simulink model "Deskrealtime"  (R2019b)
settings: Solver=FixedStepDiscrete  StartTime=0.0  StopTime=200  FixedStep=0.1  RelTol=1e-3  AbsTol=1e-6
model workspace (MATLAB code in the model file + MAT data in the model file):
  | Ts=0.1;
undefined symbols (not defined in the file or in its folder): National_Instruments, PCIe, sldrtexcb_modeswitch
libraries: xpcseriallib x60, sldrtlib x6, xpcrtudplib x2
Description:
  | Frequency Measurement
  | 
  | The example model "sldrtex_counter" shows how to measure input signal frequency using
  | Simulink Desktop Real-Time(TM). The measured signal is connected to the counter
  | input of your data acquisition board. Counter Input block is configured
  | to reset counter each sample-hit after counter read. Dividing counter
  | value by sample time gives input signal frequency.
  | 
  | How to run this model in Normal Mode:
  | 
  | 1) Open the Counter Input block and select your data acquisition board.
  |    If there's no board installed, install it using the Install new board button.
  | 2) Double-click the orange button to switch to Normal Mode if needed.
  | 3) Start the real-time execution using Simulation->Run.
  | 
  | How to run this model in External Mode:
  | 
  | 1) Open the Counter Input block and select your data acquisition board.
  |    If there's no board installed, install it using the Install new board button.
  | 2) Double-click the orange button to switch to External Mode if needed.
  | 3) Start the real-time execution using Simulation->Run. The model will automatically
  |    build, connect to Simulink in External Mode and start.
  | 
  | Note: To run this model, you must have a data acquisition board with counter input
  |    connected to your computer.
settings Model: xpc_rtwmakecfg_data=_xpcnblib__xpcetherlib__xpcether8255xlib__xpcetherGbElib__xpciplib_  PacingRate=0.400000  Creator=The MathWorks, Inc.  LastModifiedBy=qzlab
settings SolverCC: AutoScaleAbsTol=off
settings DataIOCC: ExternalInput=[]  InitialState=[]  MaxDataPoints=5000  SaveFormat=Array  SaveOutput=off  SaveTime=off  ReturnWorkspaceOutputs=off  SignalLoggingName=sigsOut
settings OptimizationCC: BlockReduction=off  BooleanDataType=off  ExpressionDepthLimit=2147483647  InitFltsAndDblsToZero=on  EfficientMapNaN2IntZero=off  LifeSpan=inf
settings DebuggingCC: UnderspecifiedInitializationDetection=Classic  MergeDetectMultiDrivingBlocksExec=none  SignalResolutionControl=TryResolveAllWithWarning  MultiTaskDSMMsg=warning  MultiTaskCondExecSysMsg=none  IntegerOverflowMsg=none  FcnCallInpInsideContextMsg=warning  AllowSymbolicDim=off  StateNameClashWarn=warning  SymbolicDimsDataTypeCodeGenerationDiagnostic=none  SFUnexpectedBacktrackingDiag=warning  SFNoUnconditionalDefaultTransitionDiag=warning  SFExecutionAtInitializationDiag=none  IntegerSaturationMsg=none  ArithmeticOperatorsInVariantConditions=warning
settings HardwareCC: TargetBitPerLong=64  TargetBitPerPointer=64  TargetBitPerSizeT=64  TargetBitPerPtrDiffT=64  TargetIntDivRoundTo=Zero  TargetEndianess=LittleEndian  TargetWordSize=64  TargetHWDeviceType=Intel->x86-64
settings ModelReferenceCC: PropagateSignalLabelsOutOfModel=off
settings SFSimCC: SimUseLocalCustomCode=off
settings RTWCC: Description=Simulink Desktop Real-Time  SystemTargetFile=sldrt.tlc  TemplateMakefile=sldrt.tmf  RTWUseLocalCustomCode=off  RTWCompilerOptimization=on
settings CodeAppCC: MaxIdLength=95  StateflowObjectComments=on
settings SimulinkDesktopRealTimeCC: TargetPreCompLibLocation=C:\Matalb2019B\toolbox\sldrt\lib\win64  TargetLangStandard=C89/C90 (ANSI)  GeneratePreprocessorConditionals=Disable all  SupportVariableSizeSignals=off  PreserveStateflowLocalDataDimensions=off
settings ConfigComp: CovMetricSettings=d  CovHtmlReporting=on  CovSaveCumulativeToWorkspaceVar=on  CovSaveSingleToWorkspaceVar=on  CovShowResultsExplorer=off  CovExternalEMLEnable=off  CovSFcnEnable=off

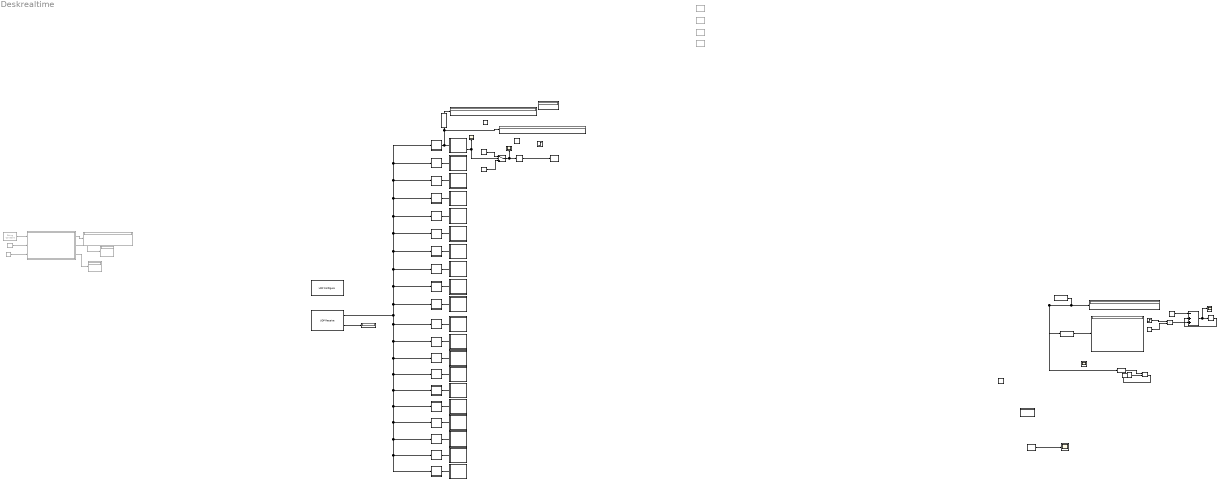
== system Deskrealtime ==
  note: Copyright 1994-2019 The MathWorks, Inc.
  note: To run the example in Normal mode, use the SIMULATION tab.
      | To run the example in External mode, use the DESKTOP REAL-TIME tab.
  1 : Subsystem
  10 : Subsystem
  11 : Subsystem
  12 : Subsystem
  13 : Subsystem
  14 : Subsystem
  15 : Subsystem
  16 : Subsystem
  17 : Subsystem
  18 : Subsystem
  19 : Subsystem
  2 : Subsystem
  2-1 : Subsystem
  2-10 : Subsystem
  2-11 : Subsystem
  2-12 : Subsystem
  2-13 : Subsystem
  2-14 : Subsystem
  2-15 : Subsystem
  2-16 : Subsystem
  2-17 : Subsystem
  2-18 : Subsystem
  2-19 : Subsystem
  2-2 : Subsystem
  2-20 : Subsystem
  2-3 : Subsystem
  2-4 : Subsystem
  2-5 : Subsystem
  2-6 : Subsystem
  2-7 : Subsystem
  2-8 : Subsystem
  2-9 : Subsystem
  20 : Subsystem
  3 : Subsystem
  4 : Subsystem
  5 : Subsystem
  6 : Subsystem
  7 : Subsystem
  8 : Subsystem
  9 : Subsystem
  ASCII to String : ASCIIToString
  ASCII to String1 : ASCIIToString
  Add : Sum  Inputs=-++
  Constant : Constant  Value=0
  Constant1 : Constant  Value=0
  Constant2 : Constant
  Constant3 : Constant
  Constant5 : Constant  Value=6  OutDataTypeStr=uint32
  Constant6 : Constant  Commented=on  Value=3  OutDataTypeStr=uint32
  Constant7 : Constant  Commented=on  OutDataTypeStr=uint32
  Constant8 : Constant
  Constant9 : Constant  Value=3
  Data Store Memory : DataStoreMemory  ReadBeforeWriteMsg=warning  WriteAfterWriteMsg=warning  WriteAfterReadMsg=warning  ShowAdditionalParam=off  OutDataTypeStr=uint32
  Data Store Write : DataStoreWrite
  Delay : Delay  DelayLength=1  InitialCondition=0
  Digital Output : sldrtlib/Digital Output  SampleTime=0.1  MaxMissedTicks=10  ShowMissedTicks=off  YieldWhenWaiting=off  DrvName=National_Instruments/PCIe-6259  DrvAddress=4294967295  DrvOptions=[0 2097151 65535 0 0]  Channels=[18:20]  BitMode=1  InitialValue=[]  FinalValue=[]
      settings: AttributesFormatString=National Instruments\nPCIe-6259 [auto]  SourceProductName=Simulink Desktop Real-Time  SourceProductBaseCode=WT
  Digital Output{1..4} (4 alike) : sldrtlib/Digital Output  Commented=on  SampleTime=0.1  MaxMissedTicks=10  ShowMissedTicks=off  YieldWhenWaiting=off  DrvName=National_Instruments/PCIe-6259  DrvAddress=4294967295  DrvOptions=[0 2097151 65535 0 0]  Channels=[19:20]  BitMode=1  InitialValue=[]  FinalValue=[]
      settings: AttributesFormatString=National Instruments\nPCIe-6259 [auto]  SourceProductName=Simulink Desktop Real-Time  SourceProductBaseCode=WT
  Display{1..3,6,8,10} (6 alike) : Display
  Display11 : Display  Commented=on
  Display12 : Display  Commented=on
  Display14 : Display  Commented=on
  Divide : Product  Inputs=*/  OutDataTypeStr=uint32
  Info : Subsystem  InitFcn=sldrtexcb_modeswitch('CheckKernel');  mask(Simulink Desktop Real-Time Example Info){}
      settings: OpenFcn=helpview([docroot '/sldrt/helptargets.map'], 'FrequencyMeasurementExample')
      mask Display: disp('Info')
  Missed Ticks : Scope
  Product : Product
  Real-Time Synchronization : sldrtlib/Real-Time Synchronization  SampleTime=0.1  MaxMissedTicks=Inf  ShowMissedTicks=on  YieldWhenWaiting=off
  Scope{,1..3} (4 alike) : Scope
  Step : Step  Time=0.01  Before=1  After=0
  Step1 : Step
  String Constant1 : StringConstant  Commented=on  String="\"123456789\""
  String Length1 : StringLength
  String to ASCII : StringToASCII
  Switch : Switch  Criteria=u2 > Threshold  Threshold=0.5
  Transport Delay : TransportDelay  DelayTime=10  InitialOutput=1
  UDP Configure : xpcrtudplib/UDP Configure  Priority=-1  IpAddress=127.0.0.1  SubnetMask=255.255.255.0  Gateway=0.0.0.0  PciBus=[2]  PciSlot=[0]  PciFunction=0  ID=1  tune=0  disable=off  enableMulticast=off  MulticastIpAddress={}  MulticastMask={}
      settings: SourceProductName=Simulink Real-Time  SourceProductBaseCode=XP
  UDP Receive2 : xpcrtudplib/UDP Receive  ipAddressVal=127.0.0.1  localPort=8001  rcvWidth=200  rcvFmAny=on  fmAddress=0.0.0.0  rcvMulticast=off  multicastAddress={}  maxUDPQueue=8  sampleTime=0.1
      settings: SourceProductName=Simulink Real-Time
  While Iterator Subsystem1 : Subsystem  Commented=on  TreatAsAtomicUnit=on
  wires:
  ASCII to String1/1 -> String to ASCII/1, String Length1/1, Display8/1
  String Length1/1 -> Divide/1
  Divide/1 -> Data Store Write/1
  Constant5/1 -> Divide/2
  String to ASCII/1 -> Display10/1
  String Constant1/1 -> While Iterator Subsystem1/1(In1)
  Constant6/1 -> While Iterator Subsystem1/2(In2)
  Constant7/1 -> While Iterator Subsystem1/3(In3)
  While Iterator Subsystem1/2(Out2) -> Display12/1
  While Iterator Subsystem1/1(Out1) -> Display11/1
  Product/1 -> Add/3
  Delay/1 -> Add/2
  Add/1 -> Scope2/1, Delay/1
  Constant8/1 -> Add/1
  Step/1 -> Product/1
  Constant9/1 -> Product/2
  While Iterator Subsystem1/3(Out3) -> Display14/1
  UDP Receive2/2 -> Display1/1
  Real-Time Synchronization/1 -> Missed Ticks/1
  UDP Receive2/1 -> 20/1(In1), 19/1(In1), 18/1(In1), 17/1(In1), 16/1(In1), 15/1(In1), 14/1(In1), 13/1(In1), 12/1(In1), 11/1(In1), 10/1(In1), 9/1(In1), 8/1(In1), 7/1(In1), 6/1(In1), 5/1(In1), 4/1(In1), 3/1(In1), 2/1(In1), 1/1(In1)
  3/1(Out1) -> 2-3/1(In1)
  2/1(Out1) -> 2-2/1(In1)
  4/1(Out1) -> 2-4/1(In1)
  5/1(Out1) -> 2-5/1(In1)
  6/1(Out1) -> 2-6/1(In1)
  7/1(Out1) -> 2-7/1(In1)
  8/1(Out1) -> 2-8/1(In1)
  9/1(Out1) -> 2-9/1(In1)
  10/1(Out1) -> 2-10/1(In1)
  11/1(Out1) -> 2-11/1(In1)
  12/1(Out1) -> 2-12/1(In1)
  13/1(Out1) -> 2-13/1(In1)
  14/1(Out1) -> 2-14/1(In1)
  15/1(Out1) -> 2-15/1(In1)
  16/1(Out1) -> 2-16/1(In1)
  17/1(Out1) -> 2-17/1(In1)
  18/1(Out1) -> 2-18/1(In1)
  19/1(Out1) -> 2-19/1(In1)
  20/1(Out1) -> 2-20/1(In1)
  2-1/3(Property) -> Scope3/1, Switch/2
  ASCII to String/1 -> Display2/1
  1/1(Out1) -> 2-1/1(In1), Display3/1, ASCII to String/1
  Constant1/1 -> Switch/1
  Switch/1 -> Transport Delay/1, Scope1/1
  Constant3/1 -> Switch/3
  Transport Delay/1 -> Digital Output/1

== system Deskrealtime/1 ==
  In1 : Inport
  ASCII to String : ASCIIToString  Commented=on
  Constant1 : Constant  Value=[1:9]
  Selector : Selector  InputPortWidth=200  IndexOptions=Index vector (port)  Indices=[1 3]  OutputSizes=1
  Out1 : Outport
  wires:
  Constant1/1 -> Selector/2
  In1/1 -> Selector/1
  Selector/1 -> Out1/1

== system Deskrealtime/10 ==
  In1 : Inport
  Constant1 : Constant  Value=[80:88]
  Selector : Selector  InputPortWidth=200  IndexOptions=Index vector (port)  Indices=[1 3]  OutputSizes=1
  Out1 : Outport
  wires:
  Constant1/1 -> Selector/2
  In1/1 -> Selector/1
  Selector/1 -> Out1/1

== system Deskrealtime/11 ==
  In1 : Inport
  Constant1 : Constant  Value=[89:89+8]
  Selector : Selector  InputPortWidth=200  IndexOptions=Index vector (port)  Indices=[1 3]  OutputSizes=1
  Out1 : Outport
  wires:
  Constant1/1 -> Selector/2
  In1/1 -> Selector/1
  Selector/1 -> Out1/1

== system Deskrealtime/12 ==
  In1 : Inport
  Constant1 : Constant  Value=[97:97+8]
  Selector : Selector  InputPortWidth=200  IndexOptions=Index vector (port)  Indices=[1 3]  OutputSizes=1
  Out1 : Outport
  wires:
  Constant1/1 -> Selector/2
  In1/1 -> Selector/1
  Selector/1 -> Out1/1

== system Deskrealtime/13 ==
  In1 : Inport
  Constant1 : Constant  Value=[105:105+8]
  Selector : Selector  InputPortWidth=200  IndexOptions=Index vector (port)  Indices=[1 3]  OutputSizes=1
  Out1 : Outport
  wires:
  Constant1/1 -> Selector/2
  In1/1 -> Selector/1
  Selector/1 -> Out1/1

== system Deskrealtime/14 ==
  In1 : Inport
  Constant1 : Constant  Value=[114:122]
  Selector : Selector  InputPortWidth=200  IndexOptions=Index vector (port)  Indices=[1 3]  OutputSizes=1
  Out1 : Outport
  wires:
  Constant1/1 -> Selector/2
  In1/1 -> Selector/1
  Selector/1 -> Out1/1

== system Deskrealtime/15 ==
  In1 : Inport
  Constant1 : Constant  Value=[123:123+8]
  Selector : Selector  InputPortWidth=200  IndexOptions=Index vector (port)  Indices=[1 3]  OutputSizes=1
  Out1 : Outport
  wires:
  Selector/1 -> Out1/1
  In1/1 -> Selector/1
  Constant1/1 -> Selector/2

== system Deskrealtime/16 ==
  In1 : Inport
  Constant1 : Constant  Value=[132:132+8]
  Selector : Selector  InputPortWidth=200  IndexOptions=Index vector (port)  Indices=[1 3]  OutputSizes=1
  Out1 : Outport
  wires:
  Selector/1 -> Out1/1
  In1/1 -> Selector/1
  Constant1/1 -> Selector/2

== system Deskrealtime/17 ==
  In1 : Inport
  Constant1 : Constant  Value=[141:141+8]
  Selector : Selector  InputPortWidth=200  IndexOptions=Index vector (port)  Indices=[1 3]  OutputSizes=1
  Out1 : Outport
  wires:
  Constant1/1 -> Selector/2
  In1/1 -> Selector/1
  Selector/1 -> Out1/1

== system Deskrealtime/18 ==
  In1 : Inport
  Constant1 : Constant  Value=[150:158]
  Selector : Selector  InputPortWidth=200  IndexOptions=Index vector (port)  Indices=[1 3]  OutputSizes=1
  Out1 : Outport
  wires:
  Selector/1 -> Out1/1
  In1/1 -> Selector/1
  Constant1/1 -> Selector/2

== system Deskrealtime/19 ==
  In1 : Inport
  Constant1 : Constant  Value=[159:159+8]
  Selector : Selector  InputPortWidth=200  IndexOptions=Index vector (port)  Indices=[1 3]  OutputSizes=1
  Out1 : Outport
  wires:
  Constant1/1 -> Selector/2
  In1/1 -> Selector/1
  Selector/1 -> Out1/1

== system Deskrealtime/2 ==
  In1 : Inport
  ASCII to String : ASCIIToString  Commented=on
  Constant1 : Constant  Value=[10:18]
  Selector : Selector  InputPortWidth=200  IndexOptions=Index vector (port)  Indices=[1 3]  OutputSizes=1
  Out1 : Outport
  wires:
  Constant1/1 -> Selector/2
  In1/1 -> Selector/1
  Selector/1 -> Out1/1

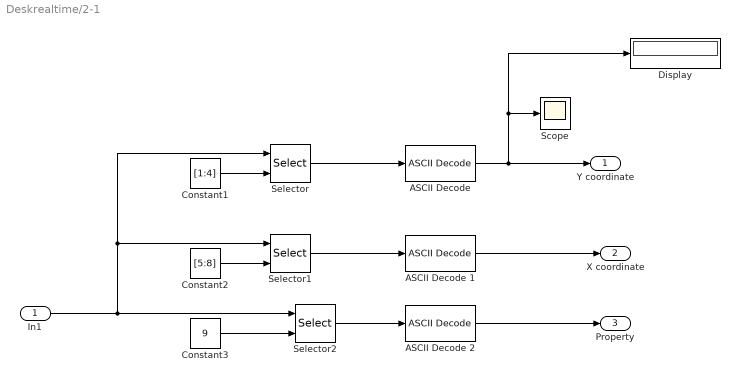
== system Deskrealtime/2-1 ==
  In1 : Inport
  "ASCII Decode " : xpcseriallib/ASCII Decode   format=%d\r  nvars=1  vartypes={ }
      settings: SourceProductName=Simulink Real-Time  SourceProductBaseCode=XP
  ASCII Decode 1 : xpcseriallib/ASCII Decode   format=%d\r  nvars=1  vartypes={ }
      settings: SourceProductName=Simulink Real-Time  SourceProductBaseCode=XP
  ASCII Decode 2 : xpcseriallib/ASCII Decode   format=%d\r  nvars=1  vartypes={ }
      settings: SourceProductName=Simulink Real-Time  SourceProductBaseCode=XP
  Constant1 : Constant  Value=[1:4]
  Constant2 : Constant  Value=[5:8]
  Constant3 : Constant  Value=9
  Display : Display
  Scope : Scope
  Selector : Selector  InputPortWidth=9  IndexOptions=Index vector (port)  Indices=[1 3]  OutputSizes=1
  Selector1 : Selector  InputPortWidth=9  IndexOptions=Index vector (port)  Indices=[1 3]  OutputSizes=1
  Selector2 : Selector  InputPortWidth=9  IndexOptions=Index vector (port)  Indices=[1 3]  OutputSizes=1
  Y coordinate : Outport
  X coordinate : Outport  Port=2
  Property : Outport  Port=3
  wires:
  Constant1/1 -> Selector/2
  In1/1 -> Selector2/1, Selector1/1, Selector/1
  Selector/1 -> "ASCII Decode "/1
  Constant2/1 -> Selector1/2
  Constant3/1 -> Selector2/2
  Selector1/1 -> ASCII Decode 1/1
  Selector2/1 -> ASCII Decode 2/1
  ASCII Decode 1/1 -> X coordinate/1
  ASCII Decode 2/1 -> Property/1
  "ASCII Decode "/1 -> Y coordinate/1, Display/1, Scope/1

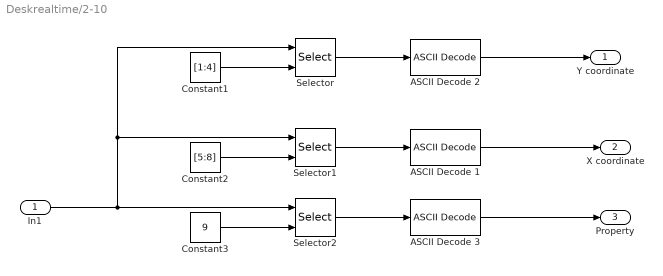
== system Deskrealtime/2-10 ==
  In1 : Inport
  ASCII Decode 1 : xpcseriallib/ASCII Decode   format=%d\r  nvars=1  vartypes={ }
      settings: SourceProductName=Simulink Real-Time  SourceProductBaseCode=XP
  ASCII Decode 2 : xpcseriallib/ASCII Decode   format=%d\r  nvars=1  vartypes={ }
      settings: SourceProductName=Simulink Real-Time  SourceProductBaseCode=XP
  ASCII Decode 3 : xpcseriallib/ASCII Decode   format=%d\r  nvars=1  vartypes={ }
      settings: SourceProductName=Simulink Real-Time  SourceProductBaseCode=XP
  Constant1 : Constant  Value=[1:4]
  Constant2 : Constant  Value=[5:8]
  Constant3 : Constant  Value=9
  Selector : Selector  InputPortWidth=9  IndexOptions=Index vector (port)  Indices=[1 3]  OutputSizes=1
  Selector1 : Selector  InputPortWidth=9  IndexOptions=Index vector (port)  Indices=[1 3]  OutputSizes=1
  Selector2 : Selector  InputPortWidth=9  IndexOptions=Index vector (port)  Indices=[1 3]  OutputSizes=1
  Y coordinate : Outport
  X coordinate : Outport  Port=2
  Property : Outport  Port=3
  wires:
  Constant1/1 -> Selector/2
  In1/1 -> Selector2/1, Selector1/1, Selector/1
  ASCII Decode 2/1 -> Y coordinate/1
  Selector/1 -> ASCII Decode 2/1
  Constant2/1 -> Selector1/2
  Constant3/1 -> Selector2/2
  Selector1/1 -> ASCII Decode 1/1
  Selector2/1 -> ASCII Decode 3/1
  ASCII Decode 1/1 -> X coordinate/1
  ASCII Decode 3/1 -> Property/1

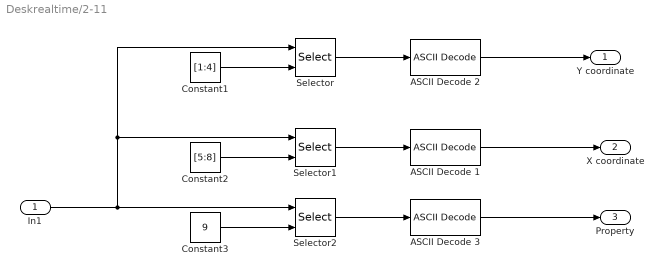
== system Deskrealtime/2-11 ==
  In1 : Inport
  ASCII Decode 1 : xpcseriallib/ASCII Decode   format=%d\r  nvars=1  vartypes={ }
      settings: SourceProductName=Simulink Real-Time  SourceProductBaseCode=XP
  ASCII Decode 2 : xpcseriallib/ASCII Decode   format=%d\r  nvars=1  vartypes={ }
      settings: SourceProductName=Simulink Real-Time  SourceProductBaseCode=XP
  ASCII Decode 3 : xpcseriallib/ASCII Decode   format=%d\r  nvars=1  vartypes={ }
      settings: SourceProductName=Simulink Real-Time  SourceProductBaseCode=XP
  Constant1 : Constant  Value=[1:4]
  Constant2 : Constant  Value=[5:8]
  Constant3 : Constant  Value=9
  Selector : Selector  InputPortWidth=9  IndexOptions=Index vector (port)  Indices=[1 3]  OutputSizes=1
  Selector1 : Selector  InputPortWidth=9  IndexOptions=Index vector (port)  Indices=[1 3]  OutputSizes=1
  Selector2 : Selector  InputPortWidth=9  IndexOptions=Index vector (port)  Indices=[1 3]  OutputSizes=1
  Y coordinate : Outport
  X coordinate : Outport  Port=2
  Property : Outport  Port=3
  wires:
  Constant1/1 -> Selector/2
  In1/1 -> Selector2/1, Selector1/1, Selector/1
  ASCII Decode 2/1 -> Y coordinate/1
  Selector/1 -> ASCII Decode 2/1
  Constant2/1 -> Selector1/2
  Constant3/1 -> Selector2/2
  Selector1/1 -> ASCII Decode 1/1
  Selector2/1 -> ASCII Decode 3/1
  ASCII Decode 1/1 -> X coordinate/1
  ASCII Decode 3/1 -> Property/1

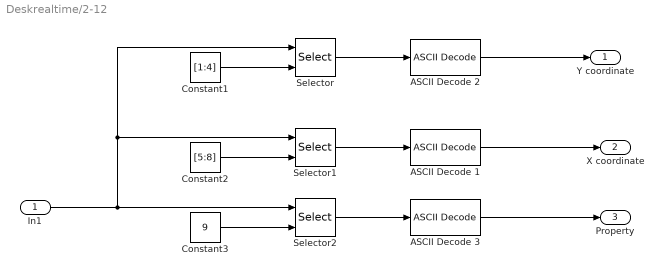
== system Deskrealtime/2-12 ==
  In1 : Inport
  ASCII Decode 1 : xpcseriallib/ASCII Decode   format=%d\r  nvars=1  vartypes={ }
      settings: SourceProductName=Simulink Real-Time  SourceProductBaseCode=XP
  ASCII Decode 2 : xpcseriallib/ASCII Decode   format=%d\r  nvars=1  vartypes={ }
      settings: SourceProductName=Simulink Real-Time  SourceProductBaseCode=XP
  ASCII Decode 3 : xpcseriallib/ASCII Decode   format=%d\r  nvars=1  vartypes={ }
      settings: SourceProductName=Simulink Real-Time  SourceProductBaseCode=XP
  Constant1 : Constant  Value=[1:4]
  Constant2 : Constant  Value=[5:8]
  Constant3 : Constant  Value=9
  Selector : Selector  InputPortWidth=9  IndexOptions=Index vector (port)  Indices=[1 3]  OutputSizes=1
  Selector1 : Selector  InputPortWidth=9  IndexOptions=Index vector (port)  Indices=[1 3]  OutputSizes=1
  Selector2 : Selector  InputPortWidth=9  IndexOptions=Index vector (port)  Indices=[1 3]  OutputSizes=1
  Y coordinate : Outport
  X coordinate : Outport  Port=2
  Property : Outport  Port=3
  wires:
  Constant1/1 -> Selector/2
  In1/1 -> Selector2/1, Selector1/1, Selector/1
  ASCII Decode 2/1 -> Y coordinate/1
  Selector/1 -> ASCII Decode 2/1
  Constant2/1 -> Selector1/2
  Constant3/1 -> Selector2/2
  Selector1/1 -> ASCII Decode 1/1
  Selector2/1 -> ASCII Decode 3/1
  ASCII Decode 1/1 -> X coordinate/1
  ASCII Decode 3/1 -> Property/1

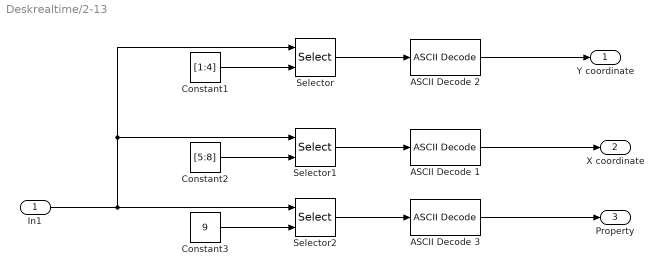
== system Deskrealtime/2-13 ==
  In1 : Inport
  ASCII Decode 1 : xpcseriallib/ASCII Decode   format=%d\r  nvars=1  vartypes={ }
      settings: SourceProductName=Simulink Real-Time  SourceProductBaseCode=XP
  ASCII Decode 2 : xpcseriallib/ASCII Decode   format=%d\r  nvars=1  vartypes={ }
      settings: SourceProductName=Simulink Real-Time  SourceProductBaseCode=XP
  ASCII Decode 3 : xpcseriallib/ASCII Decode   format=%d\r  nvars=1  vartypes={ }
      settings: SourceProductName=Simulink Real-Time  SourceProductBaseCode=XP
  Constant1 : Constant  Value=[1:4]
  Constant2 : Constant  Value=[5:8]
  Constant3 : Constant  Value=9
  Selector : Selector  InputPortWidth=9  IndexOptions=Index vector (port)  Indices=[1 3]  OutputSizes=1
  Selector1 : Selector  InputPortWidth=9  IndexOptions=Index vector (port)  Indices=[1 3]  OutputSizes=1
  Selector2 : Selector  InputPortWidth=9  IndexOptions=Index vector (port)  Indices=[1 3]  OutputSizes=1
  Y coordinate : Outport
  X coordinate : Outport  Port=2
  Property : Outport  Port=3
  wires:
  Constant1/1 -> Selector/2
  In1/1 -> Selector2/1, Selector1/1, Selector/1
  ASCII Decode 2/1 -> Y coordinate/1
  Selector/1 -> ASCII Decode 2/1
  Constant2/1 -> Selector1/2
  Constant3/1 -> Selector2/2
  Selector1/1 -> ASCII Decode 1/1
  Selector2/1 -> ASCII Decode 3/1
  ASCII Decode 1/1 -> X coordinate/1
  ASCII Decode 3/1 -> Property/1

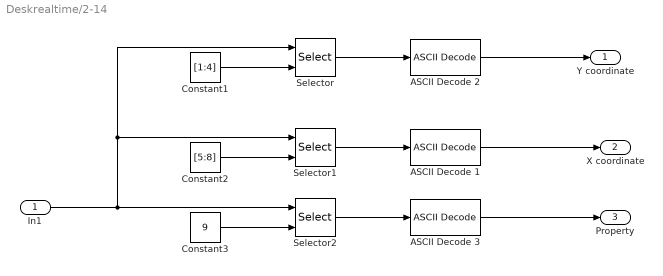
== system Deskrealtime/2-14 ==
  In1 : Inport
  ASCII Decode 1 : xpcseriallib/ASCII Decode   format=%d\r  nvars=1  vartypes={ }
      settings: SourceProductName=Simulink Real-Time  SourceProductBaseCode=XP
  ASCII Decode 2 : xpcseriallib/ASCII Decode   format=%d\r  nvars=1  vartypes={ }
      settings: SourceProductName=Simulink Real-Time  SourceProductBaseCode=XP
  ASCII Decode 3 : xpcseriallib/ASCII Decode   format=%d\r  nvars=1  vartypes={ }
      settings: SourceProductName=Simulink Real-Time  SourceProductBaseCode=XP
  Constant1 : Constant  Value=[1:4]
  Constant2 : Constant  Value=[5:8]
  Constant3 : Constant  Value=9
  Selector : Selector  InputPortWidth=9  IndexOptions=Index vector (port)  Indices=[1 3]  OutputSizes=1
  Selector1 : Selector  InputPortWidth=9  IndexOptions=Index vector (port)  Indices=[1 3]  OutputSizes=1
  Selector2 : Selector  InputPortWidth=9  IndexOptions=Index vector (port)  Indices=[1 3]  OutputSizes=1
  Y coordinate : Outport
  X coordinate : Outport  Port=2
  Property : Outport  Port=3
  wires:
  Constant1/1 -> Selector/2
  In1/1 -> Selector2/1, Selector1/1, Selector/1
  ASCII Decode 2/1 -> Y coordinate/1
  Selector/1 -> ASCII Decode 2/1
  Constant2/1 -> Selector1/2
  Constant3/1 -> Selector2/2
  Selector1/1 -> ASCII Decode 1/1
  Selector2/1 -> ASCII Decode 3/1
  ASCII Decode 1/1 -> X coordinate/1
  ASCII Decode 3/1 -> Property/1

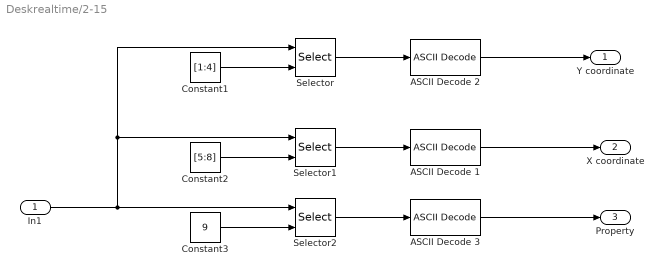
== system Deskrealtime/2-15 ==
  In1 : Inport
  ASCII Decode 1 : xpcseriallib/ASCII Decode   format=%d\r  nvars=1  vartypes={ }
      settings: SourceProductName=Simulink Real-Time  SourceProductBaseCode=XP
  ASCII Decode 2 : xpcseriallib/ASCII Decode   format=%d\r  nvars=1  vartypes={ }
      settings: SourceProductName=Simulink Real-Time  SourceProductBaseCode=XP
  ASCII Decode 3 : xpcseriallib/ASCII Decode   format=%d\r  nvars=1  vartypes={ }
      settings: SourceProductName=Simulink Real-Time  SourceProductBaseCode=XP
  Constant1 : Constant  Value=[1:4]
  Constant2 : Constant  Value=[5:8]
  Constant3 : Constant  Value=9
  Selector : Selector  InputPortWidth=9  IndexOptions=Index vector (port)  Indices=[1 3]  OutputSizes=1
  Selector1 : Selector  InputPortWidth=9  IndexOptions=Index vector (port)  Indices=[1 3]  OutputSizes=1
  Selector2 : Selector  InputPortWidth=9  IndexOptions=Index vector (port)  Indices=[1 3]  OutputSizes=1
  Y coordinate : Outport
  X coordinate : Outport  Port=2
  Property : Outport  Port=3
  wires:
  Constant1/1 -> Selector/2
  In1/1 -> Selector2/1, Selector1/1, Selector/1
  ASCII Decode 2/1 -> Y coordinate/1
  Selector/1 -> ASCII Decode 2/1
  Constant2/1 -> Selector1/2
  Constant3/1 -> Selector2/2
  Selector1/1 -> ASCII Decode 1/1
  Selector2/1 -> ASCII Decode 3/1
  ASCII Decode 1/1 -> X coordinate/1
  ASCII Decode 3/1 -> Property/1

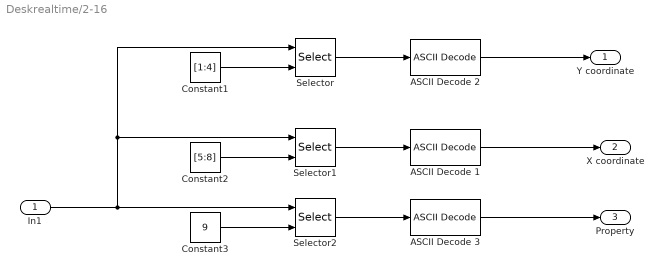
== system Deskrealtime/2-16 ==
  In1 : Inport
  ASCII Decode 1 : xpcseriallib/ASCII Decode   format=%d\r  nvars=1  vartypes={ }
      settings: SourceProductName=Simulink Real-Time  SourceProductBaseCode=XP
  ASCII Decode 2 : xpcseriallib/ASCII Decode   format=%d\r  nvars=1  vartypes={ }
      settings: SourceProductName=Simulink Real-Time  SourceProductBaseCode=XP
  ASCII Decode 3 : xpcseriallib/ASCII Decode   format=%d\r  nvars=1  vartypes={ }
      settings: SourceProductName=Simulink Real-Time  SourceProductBaseCode=XP
  Constant1 : Constant  Value=[1:4]
  Constant2 : Constant  Value=[5:8]
  Constant3 : Constant  Value=9
  Selector : Selector  InputPortWidth=9  IndexOptions=Index vector (port)  Indices=[1 3]  OutputSizes=1
  Selector1 : Selector  InputPortWidth=9  IndexOptions=Index vector (port)  Indices=[1 3]  OutputSizes=1
  Selector2 : Selector  InputPortWidth=9  IndexOptions=Index vector (port)  Indices=[1 3]  OutputSizes=1
  Y coordinate : Outport
  X coordinate : Outport  Port=2
  Property : Outport  Port=3
  wires:
  Constant1/1 -> Selector/2
  In1/1 -> Selector2/1, Selector1/1, Selector/1
  ASCII Decode 2/1 -> Y coordinate/1
  Selector/1 -> ASCII Decode 2/1
  Constant2/1 -> Selector1/2
  Constant3/1 -> Selector2/2
  Selector1/1 -> ASCII Decode 1/1
  Selector2/1 -> ASCII Decode 3/1
  ASCII Decode 1/1 -> X coordinate/1
  ASCII Decode 3/1 -> Property/1

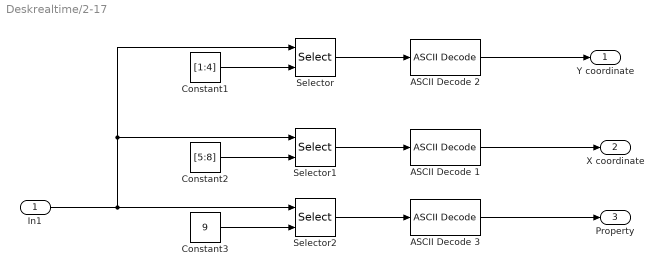
== system Deskrealtime/2-17 ==
  In1 : Inport
  ASCII Decode 1 : xpcseriallib/ASCII Decode   format=%d\r  nvars=1  vartypes={ }
      settings: SourceProductName=Simulink Real-Time  SourceProductBaseCode=XP
  ASCII Decode 2 : xpcseriallib/ASCII Decode   format=%d\r  nvars=1  vartypes={ }
      settings: SourceProductName=Simulink Real-Time  SourceProductBaseCode=XP
  ASCII Decode 3 : xpcseriallib/ASCII Decode   format=%d\r  nvars=1  vartypes={ }
      settings: SourceProductName=Simulink Real-Time  SourceProductBaseCode=XP
  Constant1 : Constant  Value=[1:4]
  Constant2 : Constant  Value=[5:8]
  Constant3 : Constant  Value=9
  Selector : Selector  InputPortWidth=9  IndexOptions=Index vector (port)  Indices=[1 3]  OutputSizes=1
  Selector1 : Selector  InputPortWidth=9  IndexOptions=Index vector (port)  Indices=[1 3]  OutputSizes=1
  Selector2 : Selector  InputPortWidth=9  IndexOptions=Index vector (port)  Indices=[1 3]  OutputSizes=1
  Y coordinate : Outport
  X coordinate : Outport  Port=2
  Property : Outport  Port=3
  wires:
  Constant1/1 -> Selector/2
  In1/1 -> Selector2/1, Selector1/1, Selector/1
  ASCII Decode 2/1 -> Y coordinate/1
  Selector/1 -> ASCII Decode 2/1
  Constant2/1 -> Selector1/2
  Constant3/1 -> Selector2/2
  Selector1/1 -> ASCII Decode 1/1
  Selector2/1 -> ASCII Decode 3/1
  ASCII Decode 1/1 -> X coordinate/1
  ASCII Decode 3/1 -> Property/1

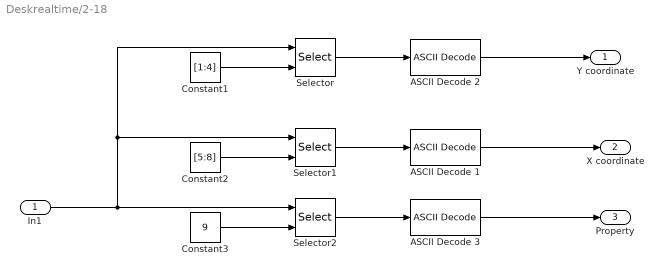
== system Deskrealtime/2-18 ==
  In1 : Inport
  ASCII Decode 1 : xpcseriallib/ASCII Decode   format=%d\r  nvars=1  vartypes={ }
      settings: SourceProductName=Simulink Real-Time  SourceProductBaseCode=XP
  ASCII Decode 2 : xpcseriallib/ASCII Decode   format=%d\r  nvars=1  vartypes={ }
      settings: SourceProductName=Simulink Real-Time  SourceProductBaseCode=XP
  ASCII Decode 3 : xpcseriallib/ASCII Decode   format=%d\r  nvars=1  vartypes={ }
      settings: SourceProductName=Simulink Real-Time  SourceProductBaseCode=XP
  Constant1 : Constant  Value=[1:4]
  Constant2 : Constant  Value=[5:8]
  Constant3 : Constant  Value=9
  Selector : Selector  InputPortWidth=9  IndexOptions=Index vector (port)  Indices=[1 3]  OutputSizes=1
  Selector1 : Selector  InputPortWidth=9  IndexOptions=Index vector (port)  Indices=[1 3]  OutputSizes=1
  Selector2 : Selector  InputPortWidth=9  IndexOptions=Index vector (port)  Indices=[1 3]  OutputSizes=1
  Y coordinate : Outport
  X coordinate : Outport  Port=2
  Property : Outport  Port=3
  wires:
  Constant1/1 -> Selector/2
  In1/1 -> Selector2/1, Selector1/1, Selector/1
  ASCII Decode 2/1 -> Y coordinate/1
  Selector/1 -> ASCII Decode 2/1
  Constant2/1 -> Selector1/2
  Constant3/1 -> Selector2/2
  Selector1/1 -> ASCII Decode 1/1
  Selector2/1 -> ASCII Decode 3/1
  ASCII Decode 1/1 -> X coordinate/1
  ASCII Decode 3/1 -> Property/1

== system Deskrealtime/2-19 ==
  In1 : Inport
  ASCII Decode 1 : xpcseriallib/ASCII Decode   format=%d\r  nvars=1  vartypes={ }
      settings: SourceProductName=Simulink Real-Time  SourceProductBaseCode=XP
  ASCII Decode 2 : xpcseriallib/ASCII Decode   format=%d\r  nvars=1  vartypes={ }
      settings: SourceProductName=Simulink Real-Time  SourceProductBaseCode=XP
  ASCII Decode 3 : xpcseriallib/ASCII Decode   format=%d\r  nvars=1  vartypes={ }
      settings: SourceProductName=Simulink Real-Time  SourceProductBaseCode=XP
  Constant1 : Constant  Value=[1:4]
  Constant2 : Constant  Value=[5:8]
  Constant3 : Constant  Value=9
  Selector : Selector  InputPortWidth=9  IndexOptions=Index vector (port)  Indices=[1 3]  OutputSizes=1
  Selector1 : Selector  InputPortWidth=9  IndexOptions=Index vector (port)  Indices=[1 3]  OutputSizes=1
  Selector2 : Selector  InputPortWidth=9  IndexOptions=Index vector (port)  Indices=[1 3]  OutputSizes=1
  Y coordinate : Outport
  X coordinate : Outport  Port=2
  Property : Outport  Port=3
  wires:
  Constant1/1 -> Selector/2
  In1/1 -> Selector2/1, Selector1/1, Selector/1
  ASCII Decode 2/1 -> Y coordinate/1
  Selector/1 -> ASCII Decode 2/1
  Constant2/1 -> Selector1/2
  Constant3/1 -> Selector2/2
  Selector1/1 -> ASCII Decode 1/1
  Selector2/1 -> ASCII Decode 3/1
  ASCII Decode 1/1 -> X coordinate/1
  ASCII Decode 3/1 -> Property/1

== system Deskrealtime/2-2 ==
  In1 : Inport
  ASCII Decode 1 : xpcseriallib/ASCII Decode   format=%d\r  nvars=1  vartypes={ }
      settings: SourceProductName=Simulink Real-Time  SourceProductBaseCode=XP
  ASCII Decode 2 : xpcseriallib/ASCII Decode   format=%d\r  nvars=1  vartypes={ }
      settings: SourceProductName=Simulink Real-Time  SourceProductBaseCode=XP
  ASCII Decode 3 : xpcseriallib/ASCII Decode   format=%d\r  nvars=1  vartypes={ }
      settings: SourceProductName=Simulink Real-Time  SourceProductBaseCode=XP
  Constant1 : Constant  Value=[1:4]
  Constant2 : Constant  Value=[5:8]
  Constant3 : Constant  Value=9
  Selector : Selector  InputPortWidth=9  IndexOptions=Index vector (port)  Indices=[1 3]  OutputSizes=1
  Selector1 : Selector  InputPortWidth=9  IndexOptions=Index vector (port)  Indices=[1 3]  OutputSizes=1
  Selector2 : Selector  InputPortWidth=9  IndexOptions=Index vector (port)  Indices=[1 3]  OutputSizes=1
  Y coordinate : Outport
  X coordinate : Outport  Port=2
  Property : Outport  Port=3
  wires:
  Constant1/1 -> Selector/2
  In1/1 -> Selector2/1, Selector1/1, Selector/1
  ASCII Decode 2/1 -> Y coordinate/1
  Selector/1 -> ASCII Decode 2/1
  Constant2/1 -> Selector1/2
  Constant3/1 -> Selector2/2
  Selector1/1 -> ASCII Decode 1/1
  Selector2/1 -> ASCII Decode 3/1
  ASCII Decode 1/1 -> X coordinate/1
  ASCII Decode 3/1 -> Property/1

== system Deskrealtime/2-20 ==
  In1 : Inport
  ASCII Decode 1 : xpcseriallib/ASCII Decode   format=%d\r  nvars=1  vartypes={ }
      settings: SourceProductName=Simulink Real-Time  SourceProductBaseCode=XP
  ASCII Decode 2 : xpcseriallib/ASCII Decode   format=%d\r  nvars=1  vartypes={ }
      settings: SourceProductName=Simulink Real-Time  SourceProductBaseCode=XP
  ASCII Decode 3 : xpcseriallib/ASCII Decode   format=%d\r  nvars=1  vartypes={ }
      settings: SourceProductName=Simulink Real-Time  SourceProductBaseCode=XP
  Constant1 : Constant  Value=[1:4]
  Constant2 : Constant  Value=[5:8]
  Constant3 : Constant  Value=9
  Selector : Selector  InputPortWidth=9  IndexOptions=Index vector (port)  Indices=[1 3]  OutputSizes=1
  Selector1 : Selector  InputPortWidth=9  IndexOptions=Index vector (port)  Indices=[1 3]  OutputSizes=1
  Selector2 : Selector  InputPortWidth=9  IndexOptions=Index vector (port)  Indices=[1 3]  OutputSizes=1
  Y coordinate : Outport
  X coordinate : Outport  Port=2
  Property : Outport  Port=3
  wires:
  Constant1/1 -> Selector/2
  In1/1 -> Selector2/1, Selector1/1, Selector/1
  ASCII Decode 2/1 -> Y coordinate/1
  Selector/1 -> ASCII Decode 2/1
  Constant2/1 -> Selector1/2
  Constant3/1 -> Selector2/2
  Selector1/1 -> ASCII Decode 1/1
  Selector2/1 -> ASCII Decode 3/1
  ASCII Decode 1/1 -> X coordinate/1
  ASCII Decode 3/1 -> Property/1

== system Deskrealtime/2-3 ==
  In1 : Inport
  ASCII Decode 1 : xpcseriallib/ASCII Decode   format=%d\r  nvars=1  vartypes={ }
      settings: SourceProductName=Simulink Real-Time  SourceProductBaseCode=XP
  ASCII Decode 2 : xpcseriallib/ASCII Decode   format=%d\r  nvars=1  vartypes={ }
      settings: SourceProductName=Simulink Real-Time  SourceProductBaseCode=XP
  ASCII Decode 3 : xpcseriallib/ASCII Decode   format=%d\r  nvars=1  vartypes={ }
      settings: SourceProductName=Simulink Real-Time  SourceProductBaseCode=XP
  Constant1 : Constant  Value=[1:4]
  Constant2 : Constant  Value=[5:8]
  Constant3 : Constant  Value=9
  Selector : Selector  InputPortWidth=9  IndexOptions=Index vector (port)  Indices=[1 3]  OutputSizes=1
  Selector1 : Selector  InputPortWidth=9  IndexOptions=Index vector (port)  Indices=[1 3]  OutputSizes=1
  Selector2 : Selector  InputPortWidth=9  IndexOptions=Index vector (port)  Indices=[1 3]  OutputSizes=1
  Y coordinate : Outport
  X coordinate : Outport  Port=2
  Property : Outport  Port=3
  wires:
  Constant1/1 -> Selector/2
  In1/1 -> Selector2/1, Selector1/1, Selector/1
  ASCII Decode 2/1 -> Y coordinate/1
  Selector/1 -> ASCII Decode 2/1
  Constant2/1 -> Selector1/2
  Constant3/1 -> Selector2/2
  Selector1/1 -> ASCII Decode 1/1
  Selector2/1 -> ASCII Decode 3/1
  ASCII Decode 1/1 -> X coordinate/1
  ASCII Decode 3/1 -> Property/1

== system Deskrealtime/2-4 ==
  In1 : Inport
  ASCII Decode 1 : xpcseriallib/ASCII Decode   format=%d\r  nvars=1  vartypes={ }
      settings: SourceProductName=Simulink Real-Time  SourceProductBaseCode=XP
  ASCII Decode 2 : xpcseriallib/ASCII Decode   format=%d\r  nvars=1  vartypes={ }
      settings: SourceProductName=Simulink Real-Time  SourceProductBaseCode=XP
  ASCII Decode 3 : xpcseriallib/ASCII Decode   format=%d\r  nvars=1  vartypes={ }
      settings: SourceProductName=Simulink Real-Time  SourceProductBaseCode=XP
  Constant1 : Constant  Value=[1:4]
  Constant2 : Constant  Value=[5:8]
  Constant3 : Constant  Value=9
  Selector : Selector  InputPortWidth=9  IndexOptions=Index vector (port)  Indices=[1 3]  OutputSizes=1
  Selector1 : Selector  InputPortWidth=9  IndexOptions=Index vector (port)  Indices=[1 3]  OutputSizes=1
  Selector2 : Selector  InputPortWidth=9  IndexOptions=Index vector (port)  Indices=[1 3]  OutputSizes=1
  Y coordinate : Outport
  X coordinate : Outport  Port=2
  Property : Outport  Port=3
  wires:
  Constant1/1 -> Selector/2
  In1/1 -> Selector2/1, Selector1/1, Selector/1
  ASCII Decode 2/1 -> Y coordinate/1
  Selector/1 -> ASCII Decode 2/1
  Constant2/1 -> Selector1/2
  Constant3/1 -> Selector2/2
  Selector1/1 -> ASCII Decode 1/1
  Selector2/1 -> ASCII Decode 3/1
  ASCII Decode 1/1 -> X coordinate/1
  ASCII Decode 3/1 -> Property/1

== system Deskrealtime/2-5 ==
  In1 : Inport
  ASCII Decode 1 : xpcseriallib/ASCII Decode   format=%d\r  nvars=1  vartypes={ }
      settings: SourceProductName=Simulink Real-Time  SourceProductBaseCode=XP
  ASCII Decode 2 : xpcseriallib/ASCII Decode   format=%d\r  nvars=1  vartypes={ }
      settings: SourceProductName=Simulink Real-Time  SourceProductBaseCode=XP
  ASCII Decode 3 : xpcseriallib/ASCII Decode   format=%d\r  nvars=1  vartypes={ }
      settings: SourceProductName=Simulink Real-Time  SourceProductBaseCode=XP
  Constant1 : Constant  Value=[1:4]
  Constant2 : Constant  Value=[5:8]
  Constant3 : Constant  Value=9
  Selector : Selector  InputPortWidth=9  IndexOptions=Index vector (port)  Indices=[1 3]  OutputSizes=1
  Selector1 : Selector  InputPortWidth=9  IndexOptions=Index vector (port)  Indices=[1 3]  OutputSizes=1
  Selector2 : Selector  InputPortWidth=9  IndexOptions=Index vector (port)  Indices=[1 3]  OutputSizes=1
  Y coordinate : Outport
  X coordinate : Outport  Port=2
  Property : Outport  Port=3
  wires:
  Constant1/1 -> Selector/2
  In1/1 -> Selector2/1, Selector1/1, Selector/1
  ASCII Decode 2/1 -> Y coordinate/1
  Selector/1 -> ASCII Decode 2/1
  Constant2/1 -> Selector1/2
  Constant3/1 -> Selector2/2
  Selector1/1 -> ASCII Decode 1/1
  Selector2/1 -> ASCII Decode 3/1
  ASCII Decode 1/1 -> X coordinate/1
  ASCII Decode 3/1 -> Property/1

== system Deskrealtime/2-6 ==
  In1 : Inport
  ASCII Decode 1 : xpcseriallib/ASCII Decode   format=%d\r  nvars=1  vartypes={ }
      settings: SourceProductName=Simulink Real-Time  SourceProductBaseCode=XP
  ASCII Decode 2 : xpcseriallib/ASCII Decode   format=%d\r  nvars=1  vartypes={ }
      settings: SourceProductName=Simulink Real-Time  SourceProductBaseCode=XP
  ASCII Decode 3 : xpcseriallib/ASCII Decode   format=%d\r  nvars=1  vartypes={ }
      settings: SourceProductName=Simulink Real-Time  SourceProductBaseCode=XP
  Constant1 : Constant  Value=[1:4]
  Constant2 : Constant  Value=[5:8]
  Constant3 : Constant  Value=9
  Selector : Selector  InputPortWidth=9  IndexOptions=Index vector (port)  Indices=[1 3]  OutputSizes=1
  Selector1 : Selector  InputPortWidth=9  IndexOptions=Index vector (port)  Indices=[1 3]  OutputSizes=1
  Selector2 : Selector  InputPortWidth=9  IndexOptions=Index vector (port)  Indices=[1 3]  OutputSizes=1
  Y coordinate : Outport
  X coordinate : Outport  Port=2
  Property : Outport  Port=3
  wires:
  Constant1/1 -> Selector/2
  In1/1 -> Selector2/1, Selector1/1, Selector/1
  ASCII Decode 2/1 -> Y coordinate/1
  Selector/1 -> ASCII Decode 2/1
  Constant2/1 -> Selector1/2
  Constant3/1 -> Selector2/2
  Selector1/1 -> ASCII Decode 1/1
  Selector2/1 -> ASCII Decode 3/1
  ASCII Decode 1/1 -> X coordinate/1
  ASCII Decode 3/1 -> Property/1

== system Deskrealtime/2-7 ==
  In1 : Inport
  ASCII Decode 1 : xpcseriallib/ASCII Decode   format=%d\r  nvars=1  vartypes={ }
      settings: SourceProductName=Simulink Real-Time  SourceProductBaseCode=XP
  ASCII Decode 2 : xpcseriallib/ASCII Decode   format=%d\r  nvars=1  vartypes={ }
      settings: SourceProductName=Simulink Real-Time  SourceProductBaseCode=XP
  ASCII Decode 3 : xpcseriallib/ASCII Decode   format=%d\r  nvars=1  vartypes={ }
      settings: SourceProductName=Simulink Real-Time  SourceProductBaseCode=XP
  Constant1 : Constant  Value=[1:4]
  Constant2 : Constant  Value=[5:8]
  Constant3 : Constant  Value=9
  Selector : Selector  InputPortWidth=9  IndexOptions=Index vector (port)  Indices=[1 3]  OutputSizes=1
  Selector1 : Selector  InputPortWidth=9  IndexOptions=Index vector (port)  Indices=[1 3]  OutputSizes=1
  Selector2 : Selector  InputPortWidth=9  IndexOptions=Index vector (port)  Indices=[1 3]  OutputSizes=1
  Y coordinate : Outport
  X coordinate : Outport  Port=2
  Property : Outport  Port=3
  wires:
  Constant1/1 -> Selector/2
  In1/1 -> Selector2/1, Selector1/1, Selector/1
  ASCII Decode 2/1 -> Y coordinate/1
  Selector/1 -> ASCII Decode 2/1
  Constant2/1 -> Selector1/2
  Constant3/1 -> Selector2/2
  Selector1/1 -> ASCII Decode 1/1
  Selector2/1 -> ASCII Decode 3/1
  ASCII Decode 1/1 -> X coordinate/1
  ASCII Decode 3/1 -> Property/1

== system Deskrealtime/2-8 ==
  In1 : Inport
  ASCII Decode 1 : xpcseriallib/ASCII Decode   format=%d\r  nvars=1  vartypes={ }
      settings: SourceProductName=Simulink Real-Time  SourceProductBaseCode=XP
  ASCII Decode 2 : xpcseriallib/ASCII Decode   format=%d\r  nvars=1  vartypes={ }
      settings: SourceProductName=Simulink Real-Time  SourceProductBaseCode=XP
  ASCII Decode 3 : xpcseriallib/ASCII Decode   format=%d\r  nvars=1  vartypes={ }
      settings: SourceProductName=Simulink Real-Time  SourceProductBaseCode=XP
  Constant1 : Constant  Value=[1:4]
  Constant2 : Constant  Value=[5:8]
  Constant3 : Constant  Value=9
  Selector : Selector  InputPortWidth=9  IndexOptions=Index vector (port)  Indices=[1 3]  OutputSizes=1
  Selector1 : Selector  InputPortWidth=9  IndexOptions=Index vector (port)  Indices=[1 3]  OutputSizes=1
  Selector2 : Selector  InputPortWidth=9  IndexOptions=Index vector (port)  Indices=[1 3]  OutputSizes=1
  Y coordinate : Outport
  X coordinate : Outport  Port=2
  Property : Outport  Port=3
  wires:
  Constant1/1 -> Selector/2
  In1/1 -> Selector2/1, Selector1/1, Selector/1
  ASCII Decode 2/1 -> Y coordinate/1
  Selector/1 -> ASCII Decode 2/1
  Constant2/1 -> Selector1/2
  Constant3/1 -> Selector2/2
  Selector1/1 -> ASCII Decode 1/1
  Selector2/1 -> ASCII Decode 3/1
  ASCII Decode 1/1 -> X coordinate/1
  ASCII Decode 3/1 -> Property/1

== system Deskrealtime/2-9 ==
  In1 : Inport
  ASCII Decode 1 : xpcseriallib/ASCII Decode   format=%d\r  nvars=1  vartypes={ }
      settings: SourceProductName=Simulink Real-Time  SourceProductBaseCode=XP
  ASCII Decode 2 : xpcseriallib/ASCII Decode   format=%d\r  nvars=1  vartypes={ }
      settings: SourceProductName=Simulink Real-Time  SourceProductBaseCode=XP
  ASCII Decode 3 : xpcseriallib/ASCII Decode   format=%d\r  nvars=1  vartypes={ }
      settings: SourceProductName=Simulink Real-Time  SourceProductBaseCode=XP
  Constant1 : Constant  Value=[1:4]
  Constant2 : Constant  Value=[5:8]
  Constant3 : Constant  Value=9
  Selector : Selector  InputPortWidth=9  IndexOptions=Index vector (port)  Indices=[1 3]  OutputSizes=1
  Selector1 : Selector  InputPortWidth=9  IndexOptions=Index vector (port)  Indices=[1 3]  OutputSizes=1
  Selector2 : Selector  InputPortWidth=9  IndexOptions=Index vector (port)  Indices=[1 3]  OutputSizes=1
  Y coordinate : Outport
  X coordinate : Outport  Port=2
  Property : Outport  Port=3
  wires:
  Constant1/1 -> Selector/2
  In1/1 -> Selector2/1, Selector1/1, Selector/1
  ASCII Decode 2/1 -> Y coordinate/1
  Selector/1 -> ASCII Decode 2/1
  Constant2/1 -> Selector1/2
  Constant3/1 -> Selector2/2
  Selector1/1 -> ASCII Decode 1/1
  Selector2/1 -> ASCII Decode 3/1
  ASCII Decode 1/1 -> X coordinate/1
  ASCII Decode 3/1 -> Property/1

== system Deskrealtime/20 ==
  In1 : Inport
  Constant1 : Constant  Value=[190:198]
  Selector : Selector  InputPortWidth=200  IndexOptions=Index vector (port)  Indices=[1 3]  OutputSizes=1
  Out1 : Outport
  wires:
  Selector/1 -> Out1/1
  In1/1 -> Selector/1
  Constant1/1 -> Selector/2

== system Deskrealtime/3 ==
  In1 : Inport
  ASCII to String : ASCIIToString  Commented=on
  Constant1 : Constant  Value=[19:27]
  Selector : Selector  InputPortWidth=200  IndexOptions=Index vector (port)  Indices=[1 3]  OutputSizes=1
  Out1 : Outport
  wires:
  Constant1/1 -> Selector/2
  In1/1 -> Selector/1
  Selector/1 -> Out1/1

== system Deskrealtime/4 ==
  In1 : Inport
  ASCII to String : ASCIIToString  Commented=on
  Constant1 : Constant  Value=[27:27+8]
  Selector : Selector  InputPortWidth=200  IndexOptions=Index vector (port)  Indices=[1 3]  OutputSizes=1
  Out1 : Outport
  wires:
  Constant1/1 -> Selector/2
  In1/1 -> Selector/1
  Selector/1 -> Out1/1

== system Deskrealtime/5 ==
  In1 : Inport
  ASCII to String : ASCIIToString  Commented=on
  Constant1 : Constant  Value=[36:36+8]
  Selector : Selector  InputPortWidth=200  IndexOptions=Index vector (port)  Indices=[1 3]  OutputSizes=1
  Out1 : Outport
  wires:
  Constant1/1 -> Selector/2
  In1/1 -> Selector/1
  Selector/1 -> Out1/1

== system Deskrealtime/6 ==
  In1 : Inport
  ASCII to String : ASCIIToString  Commented=on
  Constant1 : Constant  Value=[45:45+8]
  Selector : Selector  InputPortWidth=200  IndexOptions=Index vector (port)  Indices=[1 3]  OutputSizes=1
  Out1 : Outport
  wires:
  Constant1/1 -> Selector/2
  In1/1 -> Selector/1
  Selector/1 -> Out1/1

== system Deskrealtime/7 ==
  In1 : Inport
  Constant1 : Constant  Value=[53:53+8]
  Selector : Selector  InputPortWidth=200  IndexOptions=Index vector (port)  Indices=[1 3]  OutputSizes=1
  Out1 : Outport
  wires:
  Constant1/1 -> Selector/2
  In1/1 -> Selector/1
  Selector/1 -> Out1/1

== system Deskrealtime/8 ==
  In1 : Inport
  Constant1 : Constant  Value=[62:70]
  Selector : Selector  InputPortWidth=200  IndexOptions=Index vector (port)  Indices=[1 3]  OutputSizes=1
  Out1 : Outport
  wires:
  Constant1/1 -> Selector/2
  In1/1 -> Selector/1
  Selector/1 -> Out1/1

== system Deskrealtime/9 ==
  In1 : Inport
  Constant1 : Constant  Value=[71:79]
  Selector : Selector  InputPortWidth=200  IndexOptions=Index vector (port)  Indices=[1 3]  OutputSizes=1
  Out1 : Outport
  wires:
  Constant1/1 -> Selector/2
  In1/1 -> Selector/1
  Selector/1 -> Out1/1

== system Deskrealtime/Info ==

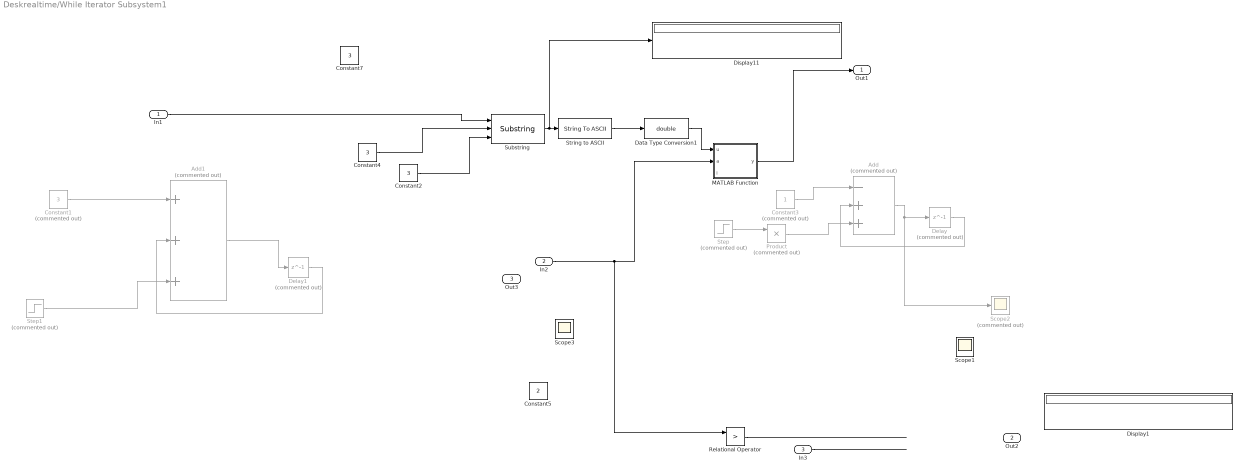
== system Deskrealtime/While Iterator Subsystem1 ==
  In1 : Inport
  In2 : Inport  Port=2
  In3 : Inport  Port=3
  Add : Sum  Commented=on  Inputs=-++
  Add1 : Sum  Commented=on  Inputs=+++
  Constant1 : Constant  Commented=on  Value=3  OutDataTypeStr=int8
  Constant2 : Constant  Value=3  OutDataTypeStr=uint8
  Constant3 : Constant  Commented=on
  Constant4 : Constant  Value=3  OutDataTypeStr=uint8
  Constant5 : Constant  Value=2  OutDataTypeStr=uint8
  Constant7 : Constant  Value=3  OutDataTypeStr=uint8
  Data Type Conversion1 : DataTypeConversion  OutDataTypeStr=double
  Delay : Delay  Commented=on  DelayLength=1  InitialCondition=0
  Delay1 : Delay  Commented=on  DelayLength=1  InitialCondition=0
  Display1 : Display
  Display11 : Display
  MATLAB Function : MATLAB Function  TreatAsAtomicUnit=on
  Product : Product  Commented=on
  Relational Operator : RelationalOperator  Operator=>  OutDataTypeStr=boolean  RndMeth=Simplest
  Scope1 : Scope
  Scope2 : Scope  Commented=on
  Scope3 : Scope
  Step : Step  Commented=on  Time=0.01  Before=1  After=0
  Step1 : Step  Commented=on  Time=0.01  Before=-5  After=0
  String to ASCII : StringToASCII  OutputVectorSize=3
  Substring : Substring
  Out1 : Outport
  Out2 : Outport  Port=2
  Out3 : Outport  Port=3
  wires:
  Step/1 -> Product/1
  Constant3/1 -> Add/1
  Add/1 -> Scope2/1, Delay/1
  Product/1 -> Add/3
  Delay/1 -> Add/2
  In2/1 -> Relational Operator/1, MATLAB Function/2(a)
  Relational Operator/1 -> ?
  In3/1 -> ?
  Constant1/1 -> Add1/1
  Delay1/1 -> Add1/2
  Constant2/1 -> Substring/3
  In1/1 -> Substring/1
  Step1/1 -> Add1/3
  Add1/1 -> Delay1/1
  Substring/1 -> Display11/1, String to ASCII/1
  MATLAB Function/1(y) -> Out1/1
  String to ASCII/1 -> Data Type Conversion1/1
  Data Type Conversion1/1 -> MATLAB Function/1(u)
  ? -> Display1/1, Scope1/1, MATLAB Function/3(i), Relational Operator/2, Out2/1
  Constant4/1 -> Substring/2

== matlab function Deskrealtime/While Iterator Subsystem1/MATLAB Function ==
  data: y output size=[20 3]; A data_store_memory; u input; a input; i input
function y = fcn(u,a,i)
%global A
y=zeros(a,3);
%i=1;

    y(i,:)=u;
    
%    i=i+1;
%    if i>a
 %       break
%    end
%end
